simulink model "chap5_5sim"  (Simulink 8.1)
settings: Solver=ode45  StartTime=0.0  StopTime=10  RelTol=1e-3
settings Model: Creator=liujk  LastModifiedBy=liujk  ExtModeTrigMode=oneshot  ExtModeArmWhenConnect=off
settings DataIOCC: LimitDataPoints=off
settings OptimizationCC: BlockReduction=off  BooleanDataType=off  ExpressionDepthLimit=128
settings DebuggingCC: SaveWithParameterizedLinksMsg=none  SignalResolutionControl=TryResolveAllWithWarning  SolverPrmCheckMsg=none  MultiTaskDSMMsg=warning  MultiTaskCondExecSysMsg=none  FcnCallInpInsideContextMsg=EnableAllAsError  StrictBusMsg=None
settings HardwareCC: TargetUnknown=on
settings RTWCC: IncludeERTFirstTime=on

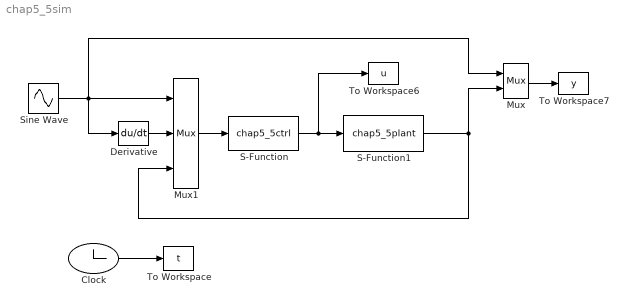
== system chap5_5sim ==
  Clock : Clock
  Derivative : Derivative
  Mux : Mux  Inputs=2
  Mux1 : Mux  Inputs=3
  S-Function : S-Function  FunctionName=chap5_5ctrl  EnableBusSupport=off
  S-Function1 : S-Function  FunctionName=chap5_5plant  EnableBusSupport=off
  Sine Wave : Sin  Frequency=pi  SampleTime=0
  To Workspace : ToWorkspace  VariableName=t  SampleTime=-1
  To Workspace6 : ToWorkspace  VariableName=u  SampleTime=-1
  To Workspace7 : ToWorkspace  VariableName=y  SampleTime=-1
  wires:
  Mux1/1 -> S-Function/1
  Mux/1 -> To Workspace7/1
  S-Function/1 -> S-Function1/1, To Workspace6/1
  Clock/1 -> To Workspace/1
  S-Function1/1 -> Mux/2, Mux1/3
  Derivative/1 -> Mux1/2
  Sine Wave/1 -> Mux/1, Mux1/1, Derivative/1
